simulink subsystem "PieroAdry"  (R2023b)
settings: Solver=VariableStepAuto  StartTime=0.0  StopTime=10.0  RelTol=1e-3
settings Model: Creator=adria  LastModifiedBy=adria

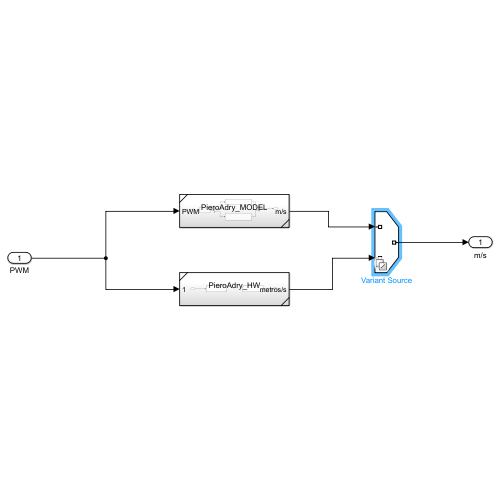
[thumbnail: Simulink's stored preview of the top-level diagram]
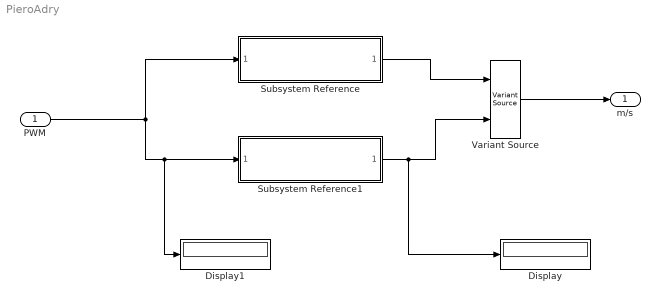
== system PieroAdry ==
  PWM : Inport
  Display : Display
  Display1 : Display
  Subsystem Reference : Subsystem  ReferencedSubsystem=PieroAdry_MODEL
  Subsystem Reference1 : Subsystem  ReferencedSubsystem=PieroAdry_HW
  Variant Source : VariantSource  VariantControlMode=sim codegen switching
  m/s : Outport
  wires:
  PWM/1 -> Subsystem Reference1/1, Display1/1, Subsystem Reference/1
  Subsystem Reference/1 -> Variant Source/1
  Variant Source/1 -> m/s/1
  Subsystem Reference1/1 -> Variant Source/2, Display/1
